simulink model "Lab8_model_2015"  (R2015a)
settings: Solver=ode15s  StartTime=0.0  StopTime=250  FixedStep=0.01  RelTol=1e-3
values from neighbouring files (symbols this model uses):
  A = pi*R1*R1    (= 10.9999393421)    [Lab2.m]    (also in ModelDataNonlinear.m)
  a = (P1y - P2y) / (P1x - P2x)    (= 0.457251908397)    [Lab4.m]    (also in Lab8.m = 0.1; Lab9.m = 0.01)
  B = (pi*R2*R2)/(3*H2*H2)    (= 0.00337009933323)    [Lab2.m]    (also in Lab8.m = deltah20max / k; Lab9.m = 0.4; ModelDataNonlinear.m)
  C1 = 1.372    [Lab2.m]    (also in ModelDataNonlinear.m)
  C2 = 0.332756    [Lab2.m]    (also in ModelDataNonlinear.m)
  deltaw = deltaq1    [Lab2.m]    (also in Lab3.m = 0; Lab8.m = deltah20max / 3; ModelDataNonlinear.m = 0.1*w0)
  h10 = (q10/C1).^2    [Lab2.m]    (also in ModelDataNonlinear.m)
  h20 = h2max/2    (= 8)    [Lab2.m]    (also in ModelDataNonlinear.m)
  kprim = -1.8    [Lab8.m]
  T1prim = 0.7    [Lab8.m]
  T2prim = 3    [Lab8.m]
  w0 = q10    [ModelDataNonlinear.m]
libraries: cstblocks x2
settings Model: Creator=Ituriello  LastModifiedBy=ishiguro
settings ConfigurationSet: Description=Simscape Multibody

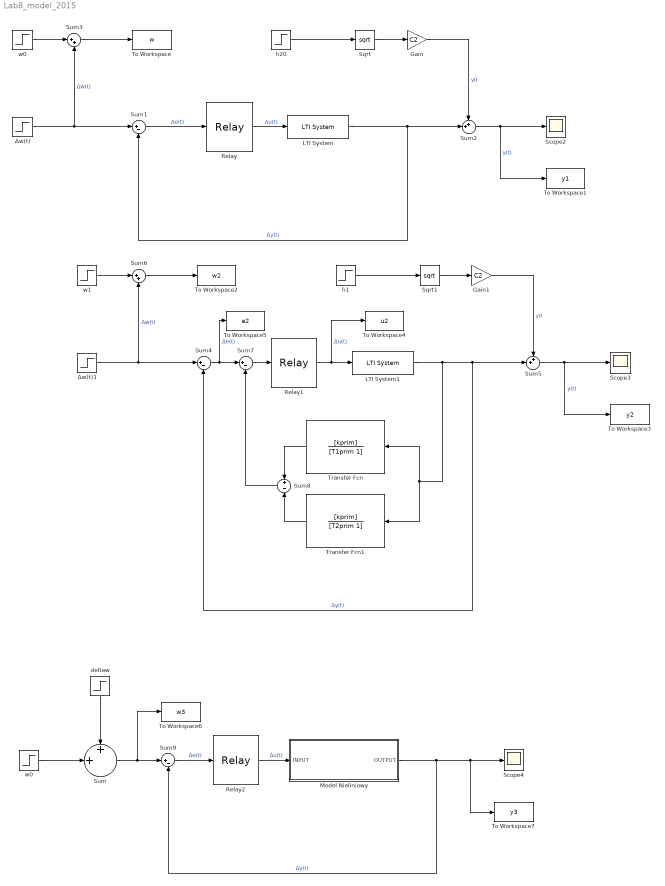
== system Lab8_model_2015 ==
  Gain : Gain  Gain=C2
  Gain1 : Gain  Gain=C2
  LTI System : cstblocks/LTI System  sys=K  IC=[]
  LTI System1 : cstblocks/LTI System  sys=K  IC=[]
  Model Nieliniowy : Subsystem
  Relay : Relay  OnSwitchValue=a  OffSwitchValue=a  OnOutputValue=B
  Relay1 : Relay  OnSwitchValue=a  OffSwitchValue=a  OnOutputValue=B
  Relay2 : Relay  OnSwitchValue=a  OffSwitchValue=a  OnOutputValue=B
  Scope2 : Scope
      settings: TimeRange=auto  LimitDataPoints=on  MaxDataPoints=5000  SaveToWorkspace=off  YMin=0.91247  YMax=1.19953  SampleTime=-1  DataFormat=Array
  Scope3 : Scope
      settings: TimeRange=auto  LimitDataPoints=on  MaxDataPoints=5000  SaveToWorkspace=off  YMin=0.91247  YMax=1.19953  SampleTime=-1  DataFormat=Array
  Scope4 : Scope
      settings: TimeRange=auto  LimitDataPoints=on  MaxDataPoints=5000  SaveToWorkspace=off  SaveName=ScopeData2  YMin=0.91247  YMax=1.19953  SampleTime=-1  DataFormat=Array
  Sqrt : Sqrt  SaturateOnIntegerOverflow=on
  Sqrt1 : Sqrt  SaturateOnIntegerOverflow=on
  Sum : Sum  Inputs=++|
  Sum{1,4,7,9} (4 alike) : Sum  Inputs=|+-
  Sum2 : Sum  Inputs=++|
  Sum3 : Sum  Inputs=|++
  Sum5 : Sum  Inputs=++|
  Sum6 : Sum  Inputs=|++
  Sum8 : Sum  Inputs=+|-
  To Workspace : ToWorkspace  VariableName=w  SaveFormat=Timeseries  SampleTime=-1
  To Workspace1 : ToWorkspace  VariableName=y1  SaveFormat=Timeseries  SampleTime=-1
  To Workspace2 : ToWorkspace  VariableName=w2  SaveFormat=Timeseries  SampleTime=-1
  To Workspace3 : ToWorkspace  VariableName=y2  SaveFormat=Timeseries  SampleTime=-1
  To Workspace4 : ToWorkspace  VariableName=u2  SaveFormat=Timeseries  SampleTime=-1
  To Workspace5 : ToWorkspace  VariableName=e2  SampleTime=-1
  To Workspace6 : ToWorkspace  VariableName=w3  SaveFormat=Timeseries  SampleTime=-1
  To Workspace7 : ToWorkspace  VariableName=y3  SaveFormat=Timeseries  SampleTime=-1
  Transfer Fcn : TransferFcn  Numerator=[kprim]  Denominator=[T1prim 1]
  Transfer Fcn1 : TransferFcn  Numerator=[kprim]  Denominator=[T2prim 1]
  deltaw : Step  Time=0  After=deltaw  SampleTime=0
  h1 : Step  Time=0  After=h20  SampleTime=0
  h20 : Step  Time=0  After=h20  SampleTime=0
  w0 : Step  Time=0  After=w0  SampleTime=0
  "w0 " : Step  Time=0  After=w0  SampleTime=0
  w1 : Step  Time=0  After=w0  SampleTime=0
  Δw(t) : Step  Time=0  After=deltaw  SampleTime=0
  Δw(t)1 : Step  Time=0  After=deltaw  SampleTime=0
  wires:
  Relay/1 -> LTI System/1  "Δu(t)"
  Sum1/1 -> Relay/1  "Δe(t)"
  LTI System/1 -> Sum2/2, Sum1/2  "Δy(t)"
  Sqrt/1 -> Gain/1
  Gain/1 -> Sum2/1  "y0"
  Sum2/1 -> To Workspace1/1, Scope2/1  "y(t)"
  h20/1 -> Sqrt/1
  Δw(t)/1 -> Sum3/2, Sum1/1  "Δw(t)"
  w0/1 -> Sum3/1
  Sum3/1 -> To Workspace/1
  "w0 "/1 -> Sum/2
  deltaw/1 -> Sum/1
  Sum6/1 -> To Workspace2/1
  Δw(t)1/1 -> Sum6/2, Sum4/1  "Δw(t)"
  w1/1 -> Sum6/1
  Relay1/1 -> To Workspace4/1, LTI System1/1  "Δu(t)"
  Sum5/1 -> To Workspace3/1, Scope3/1  "y(t)"
  h1/1 -> Sqrt1/1
  LTI System1/1 -> Transfer Fcn/1, Transfer Fcn1/1, Sum5/2, Sum4/2  "Δy(t)"
  Sqrt1/1 -> Gain1/1
  Gain1/1 -> Sum5/1  "y0"
  Sum7/1 -> Relay1/1
  Sum4/1 -> To Workspace5/1, Sum7/1  "Δe(t)"
  Sum8/1 -> Sum7/2
  Transfer Fcn/1 -> Sum8/1
  Transfer Fcn1/1 -> Sum8/2
  Relay2/1 -> Model Nieliniowy/1(INPUT)  "Δu(t)"
  Model Nieliniowy/1(OUTPUT) -> To Workspace7/1, Scope4/1, Sum9/2  "Δy(t)"
  Sum9/1 -> Relay2/1  "Δe(t)"
  Sum/1 -> To Workspace6/1, Sum9/1

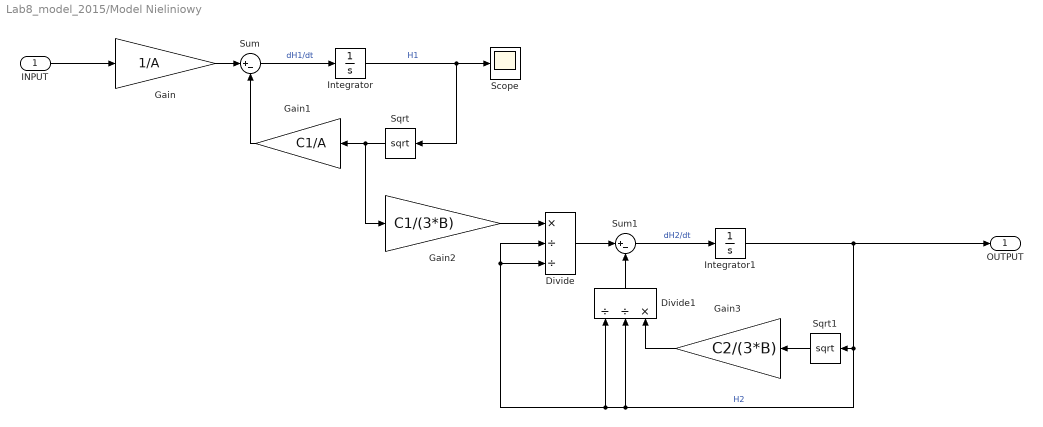
== system Lab8_model_2015/Model Nieliniowy ==
  INPUT : Inport
  Divide : Product  Inputs=*//
  Divide1 : Product  Inputs=//*
  Gain : Gain  Gain=1/A
  Gain1 : Gain  Gain=C1/A
  Gain2 : Gain  Gain=C1/(3*B)
  Gain3 : Gain  Gain=C2/(3*B)
  Integrator : Integrator  InitialCondition=h10
  Integrator1 : Integrator  InitialCondition=h20  UpperSaturationLimit=999
  Scope : Scope
      settings: TimeRange=auto  LimitDataPoints=on  MaxDataPoints=5000  SaveToWorkspace=off  SaveName=ScopeData  YMin=0.45823  YMax=0.58173  SampleTime=-1  DataFormat=Array
  Sqrt : Sqrt  SaturateOnIntegerOverflow=on
  Sqrt1 : Sqrt  SaturateOnIntegerOverflow=on
  Sum : Sum  Inputs=|+-
  Sum1 : Sum  Inputs=|+-
  OUTPUT : Outport
  wires:
  INPUT/1 -> Gain/1
  Sum/1 -> Integrator/1  "dH1/dt"
  Integrator/1 -> Sqrt/1, Scope/1  "H1"
  Sqrt/1 -> Gain2/1, Gain1/1
  Gain1/1 -> Sum/2
  Sum1/1 -> Integrator1/1  "dH2/dt"
  Sqrt1/1 -> Gain3/1
  Gain/1 -> Sum/1
  Gain3/1 -> Divide1/3
  Divide1/1 -> Sum1/2
  Divide/1 -> Sum1/1
  Gain2/1 -> Divide/1
  Integrator1/1 -> OUTPUT/1, Sqrt1/1, Divide1/2, Divide1/1, Divide/3, Divide/2  "H2"
